simulink model "terrain_follower"  (R2017a)
settings: Solver=VariableStepAuto  StartTime=0.0  StopTime=65  RelTol=1e-3
values from neighbouring files (symbols this model uses):
  A_TC = mat_lo([3 7 8 5 11], [3 7 8 5 11])    [terrain_controller.m]
  B_TC = mat_lo([3 7 8 5 11], [13 14])    [terrain_controller.m]
  C_TC = mat_lo([21 25 26 23 29], [3 7 8 5 11])    [terrain_controller.m]
  D_TC = mat_lo([21 25 26 23 29], [13 14])    [terrain_controller.m]
  distance_from_ground = 40    [terrain_controller.m]
  elevator_limits = [-25-initial_elevator 25-initial_elevator]    [terrain_controller.m]
  engine_limits = [1000-initial_thrust 19000-initial_thrust]    [terrain_controller.m]
  H_elevator_den = [1 20.2]    [terrain_controller.m]
  H_elevator_num = [20.2]    [terrain_controller.m]
  H_engine_den = [1 1]    [terrain_controller.m]
  H_engine_num = [1]    [terrain_controller.m]
  initial_altitude = 1500    [terrain_controller.m]
  K = place(state_space.A, state_space.B, [p1, p2])    [controller_pitch_rate_elevator.m]    (also in pitch_rate_controller.m = place(A_SP,B_SP,[p1,p2]))
  m_to_ft = 3.28084    [terrain_controller.m]
  trimmed_altitude = altitude    (= 5000)    [terrain_controller.m]
  velocity = input('Enter the velocity for the simulation (ft/s):  ')    [FindF16Dynamics.m]    (also in accelerometer.m = 500; normal_response_wrt_acc_pos.m = 500; pitch_rate_controller.m = 300; runF16Sim.m)
settings Model: Creator=TUDelft SID  LastModifiedBy=TUDelft SID

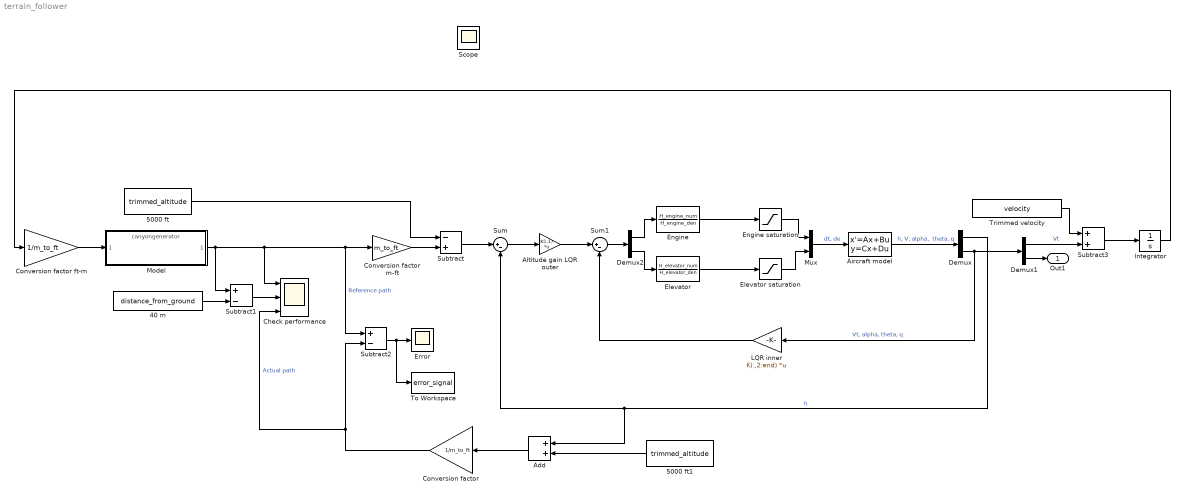
== system terrain_follower ==
  40 m : Constant  Value=distance_from_ground
  5000 ft : Constant  Value=trimmed_altitude
  5000 ft1 : Constant  Value=trimmed_altitude
  Add : Sum
  Aircraft model : StateSpace  A=A_TC  B=B_TC  C=C_TC  D=D_TC  X0=[-(trimmed_altitude - initial_altitude*m_to_ft);0; 0; 0; 0]
  Altitude gain LQR outer : Gain  Gain=K(:,1)  Multiplication=Matrix(K*u)
  Check performance : Scope  NumInputPorts=3
  "Conversion factor " : Gain  Gain=1/m_to_ft
  Conversion factor ft-m : Gain  Gain=1/m_to_ft
  Conversion factor m-ft : Gain  Gain=m_to_ft
  Demux : Demux  Outputs=[1 4]
  Demux1 : Demux  Outputs=[1 3]
  Demux2 : Demux  Outputs=[1 1]
  Elevator : TransferFcn  Numerator=H_elevator_num  Denominator=H_elevator_den
  Elevator saturation : Saturate  UpperLimit=elevator_limits(2)  LowerLimit=elevator_limits(1)
  Engine : TransferFcn  Numerator=H_engine_num  Denominator=H_engine_den
  Engine saturation : Saturate  UpperLimit=engine_limits(2)  LowerLimit=engine_limits(1)
  Error : Scope
  Integrator : Integrator
  LQR inner : Gain  Gain=K(:,2:end)  Multiplication=Matrix(K*u)
  Model : ModelReference  ModelNameDialog=canyongenerator.mdl  SimulationMode=Normal  ModelReferenceVersion=1.11
  Mux : Mux  Inputs=2
  Subtract : Sum  Inputs=-+
  Subtract1 : Sum  Inputs=+-
  Subtract2 : Sum  Inputs=+-
  Subtract3 : Sum
  Sum : Sum  Inputs=|+-
  Sum1 : Sum  Inputs=|+-
  To Workspace : ToWorkspace  VariableName=error_signal  SaveFormat=Timeseries  SampleTime=-1
  Trimmed velocity : Constant  Value=velocity
  Out1 : Outport
  Scope : Scope
  wires:
  Engine/1 -> Engine saturation/1
  Elevator/1 -> Elevator saturation/1
  Engine saturation/1 -> Mux/1
  Mux/1 -> Aircraft model/1  "dt, de"
  Elevator saturation/1 -> Mux/2
  Aircraft model/1 -> Demux/1  "h, V, alpha,  theta, q"
  Model/1 -> Subtract1/1, Check performance/1, Subtract2/1, Conversion factor m-ft/1  "Reference path"
  Subtract/1 -> Sum/1
  Demux/1 -> Add/1, Sum/2  "h"
  Demux/2 -> Demux1/1, LQR inner/1  "Vt, alpha, theta, q"
  LQR inner/1 -> Sum1/2
  Sum1/1 -> Demux2/1
  Demux2/1 -> Engine/1
  Demux2/2 -> Elevator/1
  Integrator/1 -> Conversion factor ft-m/1
  Demux1/2 -> Out1/1
  Sum/1 -> Altitude gain LQR outer/1
  Altitude gain LQR outer/1 -> Sum1/1
  Add/1 -> "Conversion factor "/1
  "Conversion factor "/1 -> Subtract2/2, Check performance/3  "Actual path"
  Conversion factor ft-m/1 -> Model/1
  Subtract2/1 -> To Workspace/1, Error/1
  Demux1/1 -> Subtract3/2  "Vt"
  Trimmed velocity/1 -> Subtract3/1
  Subtract3/1 -> Integrator/1
  40 m/1 -> Subtract1/2
  Subtract1/1 -> Check performance/2
  Conversion factor m-ft/1 -> Subtract/2
  5000 ft/1 -> Subtract/1
  5000 ft1/1 -> Add/2
